simulink model "Vector_control_10Hp_with_20usec"  (R2014a)
settings: Solver=ode5  StartTime=0.0  StopTime=10  FixedStep=20e-6  RelTol=1e-3
InitFcn:
  | Lr=0.1241+0.003045;
  | Lm=0.1241;
  | Ls=0.1241+0.003045;
undefined symbols (not defined in the file): DiscIntNeverNeededParam, driveGuiManager, gcbh, sps_rtmsupport, Ts
libraries: powerlib x10, powerlib_meascontrol x5, simulink_extras x4, AC3DriveInternalModels x2, DriveInternalModels x1, simulink x1
settings Model: Creator=Bharat  LastModifiedBy=apple
settings DebuggingCC: UnderspecifiedInitializationDetection=Classic  StateNameClashWarn=warning

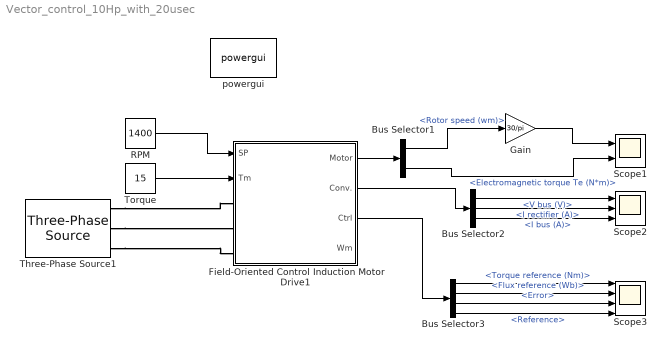
== system Vector_control_10Hp_with_20usec ==
  Bus Selector1 : BusSelector  OutputSignals=Mechanical.Rotor speed (wm),Mechanical.Electromagnetic torque Te (N*m)
  Bus Selector2 : BusSelector  OutputSignals=V bus (V),I rectifier (A),I bus (A)
  Bus Selector3 : BusSelector  OutputSignals=Torque reference (Nm),Flux reference (Wb),Error,Reference
  Field-Oriented Control Induction Motor Drive1 : Subsystem  LoadFcn=sps_rtmsupport('LoadFcn',gcbh); driveGuiManager('Load',get_param(gcb,'driveType'), gcbh);  StartFcn=sps_rtmsupport('StartFcn',gcbh);  StopFcn=|  mask(Field-Oriented Control Induction Motor Drive){showMaskWarnings=on, AverageValue=off, MechanicalLoad=Torque Tm, driveType=AC3, outputBusMode=Multiple output buses}
      | sps_rtmsupport('StopFcn',gcbh);                                   
      | %driveGuiManager('ReactivateGui',get_param(gcb,'driveType'),gcbh);
      mask prompts: showMaskWarnings "Show mask synchronization warnings"; AverageValue "Average value model"; MechanicalLoad "Mechanical input:"; driveType "Drive type"; outputBusMode "Output bus mode:"
      mask init:
      | block=gcb;
      | [X1,X1m,X2,X2m,X3,X4,Y1,Y1m,Y2,Y2m,Y3,Y4,color1,color2,INp,OUTp,Ts,machineType] = spsDrivesMaskInit(block,driveType,AverageValue);
      | %spsDrivesOutputSelectorCbak(block);
      settings: CopyFcn=sps_rtmsupport('CopyFcn',gcbh);  DeleteFcn="sps_rtmsupport('DeleteFcn',gcbh); driveGuiManager('Delete',get_param(gcb,'driveType')  ,gcbh)"  UndoDeleteFcn=sps_rtmsupport('UndoDeleteFcn',gcbh);  ModelCloseFcn=sps_rtmsupport('ModelCloseFcn',gcbh);  PreSaveFcn=sps_rtmsupport('PreSaveFcn',gcbh);  PostSaveFcn=sps_rtmsupport('PostSaveFcn',gcbh);  NameChangeFcn=sps_rtmsupport('NameChangeFcn',gcbh);  PreCopyFcn=sps_rtmsupport('PreCopyFcn',gcbh);  CloseFcn="sps_rtmsupport('CloseFcn',gcbh); %driveGuiManager('Delete',get_param(gcb,'driveType')  ,gcbh)"  PreDeleteFcn=sps_rtmsupport('PreDeleteFcn',gcbh);  ParentCloseFcn="driveGuiManager('Hide',get_param(gcb,'driveType')  ,gcbh)"
      settings: OpenFcn=|
      | sps_rtmsupport('parametereditingmodes',gcbh, [1 2 3 4 5]); if (power_openblockproxy ('secondary'))
      | driveGuiManager('Create',get_param(gcb,'driveType')  ,gcbh)
      | end;
      mask Help: helpview(psbhelp)
      mask TypeOptions MechanicalLoad: Torque Tm | Speed w | Mechanical rotational port
      mask TypeOptions driveType: AC3
      mask TypeOptions outputBusMode: Multiple output buses | Single output bus
      mask Display:
      | patch([X1 X1m],[Y1 Y1m],color1);
      | patch(X3,Y3,color2);
      | plot([X1 X1m X2 X2m X3 X4],[Y1 Y1m Y2 Y2m Y3 Y4]);
      | text(0.5,0.3,'AC3','HorizontalAlignment','center')
      | HaveSPSMec = (strcmp(MechanicalLoad,'Torque Tm') || strcmp(MechanicalLoad,'Speed w'));
      | if (HaveSPSMec==1 && strcmp(outputBusMode,'Multiple output buses'))
      |     port_label('input',2,INp)
      |     port_label('output',4,OUTp)
      | end
      | if (HaveSPSMec==1 && strcmp(outputBusMode,'Single output bus'))
      |     port_label('input',2,INp)
      |     port_label('output',2,OUTp)
      | end
  Gain : Gain  Gain=30/pi
  RPM : Constant  Value=1400
  Scope1 : Scope  NumInputPorts=2
      settings: YMin=1399.8~5  YMax=1402~20
  Scope2 : Scope  NumInputPorts=3
      settings: YMin=215~3.5~-22.5  YMax=262.5~12.5~22.5
  Scope3 : Scope  NumInputPorts=4
      settings: YMin=104.765~5.75~-5~-5  YMax=104.83~10.75~5~5  SaveName=ScopeData2
  Three-Phase Source1 : powerlib/Electrical Sources/Three-Phase Source  Voltage=400  PhaseAngle=0  Frequency=50  InternalConnection=Yg  SpecifyImpedance=on  Resistance=0.8929  Inductance=16.58e-3  ShortCircuitLevel=100e6  BaseVoltage=25e3  XRratio=7  BusType=swing  Pref=0  Qref=0  Qmin=-inf  Qmax=inf
  Torque : Constant  Value=15
  powergui : powerlib/powergui  Priority=1  SimulationMode=Discrete  SolverType=Backward Euler  SampleTime=20e-6  frequency=60  SPID=off  DisableSnubberDevices=off  DisableRonSwitches=off  DisableVfSwitches=off  SwTol=0  Interpol=off  DisplayEquations=off  Ts=0  methode=off  frequencyindice=50  Pbase=100e6  ErrMax=1e-4  Iterations=50  UnitsV=kV  UnitsW=MW  FunctionMessages=off  echomessages=off  HookPort=off  EnableUseOfTLC=off  x0status=blocks  RestoreLinks=warning  ResistiveCurrentMeasurement=off  Frange=[0:2:500]  Ylog=off  Xlog=on  ShowGrid=off  save=off  variable=ZData  structure=0  ZoomFFT=off  StartTime=0.0  cycles=1  DisplayStyle=1  fundamental=60  FreqAxis=off  MaxFrequency=1000  frequencyindicesteady=1  RmsSteady=1  display=off
  wires:
  RPM/1 -> Field-Oriented Control Induction Motor Drive1/1(SP)
  Torque/1 -> Field-Oriented Control Induction Motor Drive1/2(Tm)
  Field-Oriented Control Induction Motor Drive1/1(Motor) -> Bus Selector1/1
  Bus Selector1/1 -> Gain/1  "<Rotor speed (wm)>"
  Bus Selector1/2 -> Scope1/2  "<Electromagnetic torque Te (N*m)>"
  Field-Oriented Control Induction Motor Drive1/2(Conv.) -> Bus Selector2/1
  Bus Selector2/1 -> Scope2/1  "<V bus (V)>"
  Bus Selector2/2 -> Scope2/2  "<I rectifier (A)>"
  Field-Oriented Control Induction Motor Drive1/3(Ctrl) -> Bus Selector3/1
  Bus Selector3/1 -> Scope3/1  "<Torque reference (Nm)>"
  Bus Selector3/2 -> Scope3/2  "<Flux reference (Wb)>"
  Bus Selector2/3 -> Scope2/3  "<I bus (A)>"
  Bus Selector3/3 -> Scope3/3  "<Error>"
  Bus Selector3/4 -> Scope3/4  "<Reference>"
  Gain/1 -> Scope1/1
  connections:
  Three-Phase Source1/RConn2 -- Field-Oriented Control Induction Motor Drive1/LConn2
  Three-Phase Source1/RConn3 -- Field-Oriented Control Induction Motor Drive1/LConn3
  Three-Phase Source1/RConn1 -- Field-Oriented Control Induction Motor Drive1/LConn1

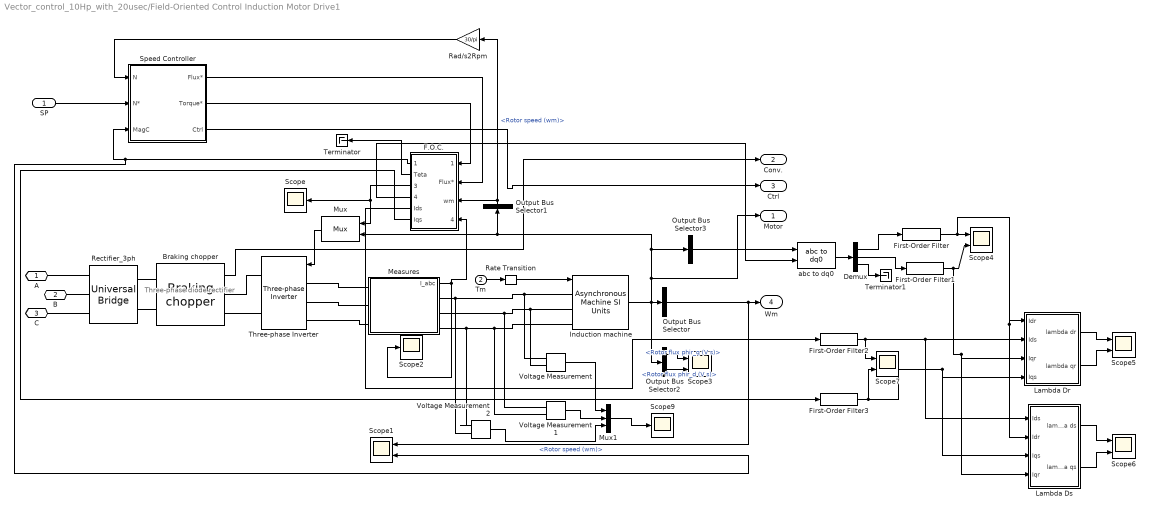
== system Vector_control_10Hp_with_20usec/Field-Oriented Control Induction Motor Drive1 ==
  note: Three-phase
      | diode rectifier
  SP : Inport
  Tm : Inport  Port=2
  Braking chopper : DriveInternalModels/AC drives/Braking chopper  chopa=500  chopd=490  freq_chop=4000  cap_bus=2000e-6  br=8
  Demux : Demux  Outputs=3
  F.O.C. : Subsystem  mask(FOC){freq_max=20000, in_flux=0.45, Lm=0.1722, Rr=1.395, Llr=0.005839, p=2, h=0.1, kp=40, ki=50, fc=16, csat=[-2,2], Tvect=20e-6}
      mask prompts: freq_max "Maximum inverter frequency (Hz)"; in_flux "Initial machine flux (Wb)"; Lm "Motor mutual inductance (H)"; Rr "Motor rotor resistance (ohms)"; Llr "Motor rotor leakage inductance (H)"; p "Motor pairs of poles"; h "Current regulator - current hysteresis bandwidth (A)"; kp "Flux controller - proportional gain"; ki "Flux controller - integral gain"; fc "Flux controller - flux estimation low-pass filter cutoff frequency (Hz)"; csat "Flux controller - controller output flux saturation (Wb) [negative,positive]"; Tvect "Vector control sampling time (s)"
      mask help: This block implements a field oriented controller.
      mask init:
      | Lr=Lm+Llr;
      | [X1,X1m,X2,X2m,X3,X4,Y1,Y1m,Y2,Y2m,Y3,Y4,color1,color2]=spsdrivelogo;
      mask Display:
      | patch([X1 X1m],[Y1 Y1m],color1);
      | patch(X3,Y3,color2);
      | plot([X1 X1m X2 X2m X3 X4],[Y1 Y1m Y2 Y2m Y3 Y4]);
  First-Order Filter : powerlib_meascontrol/Filters/First-Order Filter  FilterType=Lowpass  Tc=1/100  Ts=0  Initialize=on  Vac_Init=[0, 0, 60]  Vdc_Init=0  PlotResponse=off  FreqRange="[0,  200,  1]"
  First-Order Filter1 : powerlib_meascontrol/Filters/First-Order Filter  FilterType=Lowpass  Tc=1/100  Ts=0  Initialize=on  Vac_Init=[0, 0, 60]  Vdc_Init=0  PlotResponse=off  FreqRange="[0,  200,  1]"
  First-Order Filter2 : powerlib_meascontrol/Filters/First-Order Filter  FilterType=Lowpass  Tc=1/200  Ts=0  Initialize=on  Vac_Init=[0, 0, 60]  Vdc_Init=0  PlotResponse=off  FreqRange="[0,  200,  1]"
  First-Order Filter3 : powerlib_meascontrol/Filters/First-Order Filter  FilterType=Lowpass  Tc=1/200  Ts=0  Initialize=on  Vac_Init=[0, 0, 60]  Vdc_Init=0  PlotResponse=off  FreqRange="[0,  200,  1]"
  Induction machine : powerlib/Machines/Asynchronous Machine SI Units  PresetModel="16:  10 HP (7.5KW)  400 V 50Hz 1440 RPM"  MechanicalLoad=Torque Tm  ShowDetailedParameters=on  RotorType=Squirrel-cage  ReferenceFrame=Rotor  Units=SI  MeasurementBus=off  NominalParameters=[7500 400 50]  Stator=[0.7384 0.003045]  Rotor=[0.7402 0.003045]  Cage1=[ 0.022 0.226/377]  Cage2=[ 0.022 0.226/377]  Lm=0.1241  Mechanical=[0.0343 0.000503 2]  PolePairs=2  InitialConditions=[1,0,0,0,0,0,0,0]  SimulateSaturation=off  Saturation=[0 0;0 0]  LoadFlowParameters=0  TsPowergui=0  TsBlock=-1  IterativeModel=Forward Euler  Pmec=0
  Lambda Dr : Subsystem
  Lambda Ds : Subsystem
  Measures : Subsystem
  Mux : AC3DriveInternalModels/Mux
  Mux1 : Mux  Inputs=3
  Output Bus Selector : BusSelector  OutputSignals=Mechanical.Rotor speed (wm)
  Output Bus Selector1 : BusSelector  OutputSignals=Mechanical.Rotor speed (wm)
  Output Bus Selector2 : BusSelector  OutputSignals=Rotor measurements.Rotor flux phir_q (V s),Rotor measurements.Rotor flux phir_d (V s)
  Output Bus Selector3 : BusSelector  OutputSignals=Rotor measurements.Rotor current ir_a (A),Rotor measurements.Rotor current ir_b (A),Rotor measurements.Rotor current ir_c (A)  OutputAsBus=on
  Rad/s2Rpm : Gain  Gain=30/pi  SaturateOnIntegerOverflow=on  OutDataTypeStr=Inherit: Same as input  ParamDataTypeStr=Inherit: Same as input
  Rate Transition : RateTransition  OutPortSampleTime=Ts
  Rectifier_3ph : powerlib/Power Electronics/Universal Bridge  Arms=3  SnubberResistance=10e3  SnubberCapacitance=20e-9  Device=Diodes  Ron=1e-3  Lon=0  ForwardVoltages="[  0,  0  ]"  ForwardVoltage=1.3  GTOparameters=[ 10e-6, 20e-6 ]  IGBTparameters=[ 1e-6 , 2e-6 ]  Measurements=All voltages and currents  Measurements_2=None  converterType=Rectifier
  Scope : Scope
      settings: SaveName=ScopeData4
  Scope{1,3..7} (6 alike) : Scope  NumInputPorts=2
      Scope1 settings: YMin=32~0.95  YMax=53~1.05  SaveName=ScopeData5
      Scope3 settings: YMin=-5~-5  YMax=5~5  SaveName=ScopeData10
      Scope4 settings: YMin=0.04~-18.025  YMax=0.19~-17.825  SaveName=ScopeData11
      Scope5 settings: YMin=-2.5~-10  YMax=5~12  SaveName=ScopeData13
      Scope6 settings: YMin=-2.5~-10  YMax=5~12  SaveName=ScopeData14
      Scope7 settings: YMin=0.04~-18.025  YMax=0.19~-17.825  SaveName=ScopeData15
  Scope2 : Scope
      settings: SaveName=ScopeData8
  Scope9 : Scope
      settings: SaveName=ScopeData21
  Speed Controller : Subsystem  mask(Speed controller){SwK=Speed regulation, fn=50, ramp=[-1500,1500], kp=0.9, ki=6.4, fc=100, ctrl_sat=[-28,28], p=2, nf=0.45, Tsc=100e-6}
      mask prompts: SwK "Regulation type"; fn "Machine nominal frequency (Hz)"; ramp "Speed reference ramp  (rpm/s) [deceleration,acceleration]"; kp "Proportional gain"; ki "Integral gain"; fc "Speed measurement - low-pass filter cutoff frequency (Hz)"; ctrl_sat "Controller output torque saturation (N.m) [negative,positive]"; p "Motor pairs of poles"; nf "Machine nominal flux (Wb)"; Tsc "Controller sampling time (s)"
      mask help: This block implements a PI speed regulator.
      mask init:
      | bs=2*30*fn/p;
      | [X1,X1m,X2,X2m,X3,X4,Y1,Y1m,Y2,Y2m,Y3,Y4,color1,color2]=spsdrivelogo;
      | if SwK == 1
      |     set_param(gcb,'MaskVisibilities',{'on','on','on','on','on','on','on','on','on','on'})
      | else
      |     set_param(gcb,'MaskVisibilities',{'on','on','off','off','off','off','on','on','on','on'})
      | end
      mask TypeOptions SwK: Speed regulation | Torque regulation
      mask Display:
      | patch([X1 X1m],[Y1 Y1m],color1);
      | patch(X3,Y3,color2);
      | plot([X1 X1m X2 X2m X3 X4],[Y1 Y1m Y2 Y2m Y3 Y4]);
  Terminator : Terminator
  Terminator1 : Terminator
  Three-phase Inverter : AC3DriveInternalModels/Three-phase Inverter  Arms=3  SnubberResistance=5e3  SnubberCapacitance=inf  Device=IGBT / Diodes  Ron=1e-3  Lon=0  ForwardVoltages=[0.8,0.8]  ForwardVoltage=0  GTOparameters=[10e-6,20e-6]  IGBTParameters=[1e-6,2e-6]  Measurements=All voltages and currents  converterType=Inverter  SourceFrequency=60  Stator=[1.405,0.005839]  Rotor=[1.395,0.005839]  Lm=0.1722  p=2  ReferenceFrame=Rotor
  Voltage Measurement : powerlib/Measurements/Voltage Measurement  PhasorSimulation=off  OutputType=Complex  PSBequivalent=0
  Voltage Measurement1 : powerlib/Measurements/Voltage Measurement  PhasorSimulation=off  OutputType=Complex  PSBequivalent=0
  Voltage Measurement2 : powerlib/Measurements/Voltage Measurement  PhasorSimulation=off  OutputType=Complex  PSBequivalent=0
  abc to dq0 : powerlib_meascontrol/Transformations/abc to dq0  Alignment=Aligned with phase A axis
  A : PMIOPort  Port=1  Side=Left
  B : PMIOPort  Port=2  Side=Left
  C : PMIOPort  Port=3  Side=Left
  Motor : Outport
  Conv. : Outport  Port=2
  Ctrl : Outport  Port=3
  Wm : Outport  Port=4
  wires:
  Induction machine/1 -> Motor/1, Output Bus Selector3/1, Mux/2, Output Bus Selector1/1, Output Bus Selector2/1, Output Bus Selector/1
  Measures/1(I_abc) -> F.O.C./4(I_ABC), Scope2/1
  F.O.C./2(Teta) -> Terminator/1
  Speed Controller/3(Ctrl) -> Ctrl/1
  Speed Controller/1(Flux*) -> F.O.C./2(Flux*)
  Speed Controller/2(Torque*) -> F.O.C./1(Torque*)
  Rad/s2Rpm/1 -> Speed Controller/1(N)
  Braking chopper/1 -> Conv./1
  F.O.C./3(Gates) -> Mux/1, Scope/1
  Mux/1 -> Three-phase Inverter/1
  Output Bus Selector/1 -> Scope1/1, Wm/1  "<Rotor speed (wm)>"
  Tm/1 -> Rate Transition/1
  Rate Transition/1 -> Induction machine/1
  F.O.C./1(MagC) -> Scope1/2, Speed Controller/3(MagC)
  Output Bus Selector2/1 -> Scope3/1  "<Rotor flux phir_q (V s)>"
  Output Bus Selector2/2 -> Scope3/2  "<Rotor flux phir_d (V s)>"
  Output Bus Selector3/1 -> abc to dq0/1
  F.O.C./4(Teta1) -> abc to dq0/2
  abc to dq0/1 -> Demux/1
  Demux/1 -> First-Order Filter/1
  Demux/2 -> First-Order Filter1/1
  Demux/3 -> Terminator1/1
  First-Order Filter/1 -> Lambda Ds/2(Idr), Lambda Dr/1(Idr), Scope4/1
  First-Order Filter1/1 -> Lambda Ds/4(Iqr), Lambda Dr/3(Iqr), Scope4/2
  Lambda Dr/1(lambda dr) -> Scope5/1
  Lambda Dr/2(lambda qr) -> Scope5/2
  Lambda Ds/1(lambda ds) -> Scope6/1
  Lambda Ds/2(lambda qs) -> Scope6/2
  F.O.C./5(Ids) -> First-Order Filter2/1
  F.O.C./6(Iqs) -> First-Order Filter3/1
  First-Order Filter3/1 -> Scope7/2, Lambda Ds/3(Iqs), Lambda Dr/4(Iqs)
  First-Order Filter2/1 -> Scope7/1, Lambda Ds/1(Ids), Lambda Dr/2(Ids)
  SP/1 -> Speed Controller/2(N*)
  Voltage Measurement/1 -> Mux1/1
  Voltage Measurement1/1 -> Mux1/2
  Voltage Measurement2/1 -> Mux1/3
  Mux1/1 -> Scope9/1
  Output Bus Selector1/1 -> Rad/s2Rpm/1, F.O.C./3(wm)  "<Rotor speed (wm)>"
  connections:
  Measures/RConn1 -- Voltage Measurement2/LConn2 -- Voltage Measurement/LConn1 -- Induction machine/LConn1
  Measures/RConn2 -- Voltage Measurement1/LConn1 -- Voltage Measurement/LConn2 -- Induction machine/LConn2
  Measures/RConn3 -- Voltage Measurement2/LConn1 -- Voltage Measurement1/LConn2 -- Induction machine/LConn3
  Three-phase Inverter/LConn1 -- Measures/LConn1
  Three-phase Inverter/LConn2 -- Measures/LConn2
  Three-phase Inverter/LConn3 -- Measures/LConn3
  Braking chopper/RConn1 -- Three-phase Inverter/RConn1
  Braking chopper/RConn2 -- Three-phase Inverter/RConn2
  Braking chopper/LConn1 -- Rectifier_3ph/RConn1
  Braking chopper/LConn2 -- Rectifier_3ph/RConn2
  A/RConn1 -- Rectifier_3ph/LConn1
  B/RConn1 -- Rectifier_3ph/LConn2
  C/RConn1 -- Rectifier_3ph/LConn3

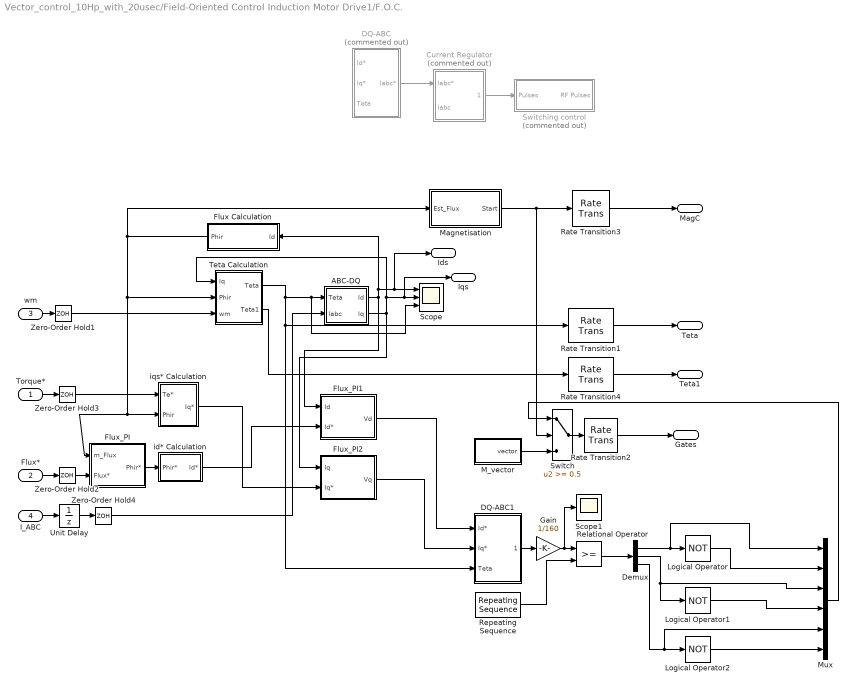
== system Vector_control_10Hp_with_20usec/Field-Oriented Control Induction Motor Drive1/F.O.C. ==
  Torque* : Inport
  Flux* : Inport  Port=2
  wm : Inport  Port=3
  I_ABC : Inport  Port=4
  ABC-DQ : Subsystem
  Current Regulator : Subsystem  Commented=on
  DQ-ABC : Subsystem  Commented=on
  DQ-ABC1 : Subsystem
  Demux : Demux  Outputs=3
  Flux Calculation : Subsystem  mask(Flux Calcultation){}
      mask init:
      | NF=0.44572610323020e-6;
      | DF=[1 -0.99998715486734];
  Flux_PI : Subsystem
  Flux_PI1 : Subsystem
  Flux_PI2 : Subsystem
  Gain : Gain  Gain=1/160
  Logical Operator : Logic  Operator=NOT  AllPortsSameDT=off  OutDataTypeStr=boolean
  Logical Operator1 : Logic  Operator=NOT  AllPortsSameDT=off  OutDataTypeStr=boolean
  Logical Operator2 : Logic  Operator=NOT  AllPortsSameDT=off  OutDataTypeStr=boolean
  M_vector : Subsystem
  Magnetisation : Subsystem
  Mux : Mux  Inputs=6
  Rate Transition1 : RateTransition  OutPortSampleTime=Ts
  Rate Transition2 : RateTransition
  Rate Transition3 : RateTransition
  Rate Transition4 : RateTransition  OutPortSampleTime=Ts
  Relational Operator : RelationalOperator  OutDataTypeStr=boolean
  Repeating Sequence : simulink/Sources/Repeating Sequence  rep_seq_t=[0 1/8000 1/4000 3/8000 1/2000]  rep_seq_y=[0 1 0 -1 0]
  Scope : Scope  NumInputPorts=3
      settings: YMin=1.5~17.5~2.5  YMax=7~22.25~35  SaveName=ScopeData3
  Scope1 : Scope
      settings: YMin=-3  YMax=3  SaveName=ScopeData12
  Switch : Switch  Threshold=0.5  SaturateOnIntegerOverflow=on
  Switching control : Subsystem  Commented=on
  Teta Calculation : Subsystem
  Unit Delay : UnitDelay  SampleTime=-1
  Zero-Order Hold{1..4} (4 alike) : ZeroOrderHold  SampleTime=Tvect
  id* Calculation : Subsystem
  iqs* Calculation : Subsystem
  MagC : Outport
  Teta : Outport  Port=2
  Gates : Outport  Port=3
  Teta1 : Outport  Port=4
  Ids : Outport  Port=5
  Iqs : Outport  Port=6
  wires:
  Zero-Order Hold2/1 -> Flux_PI/2(Flux*)
  ABC-DQ/1(Id) -> Ids/1, Scope/1, Flux Calculation/1(Id), Flux_PI1/1(Id)
  ABC-DQ/2(Iq) -> Flux_PI2/1(Iq), Teta Calculation/1(Iq), Iqs/1, Scope/2
  Flux Calculation/1(Phir) -> Magnetisation/1(Est_Flux), Teta Calculation/2(Phir), Flux_PI/1(m_Flux), iqs* Calculation/2(Phir)
  iqs* Calculation/1(Iq*) -> Flux_PI2/2(Iq*)
  id* Calculation/1(Id*) -> Flux_PI1/2(Id*)
  I_ABC/1 -> Unit Delay/1
  wm/1 -> Zero-Order Hold1/1
  Current Regulator/1(Pulses) -> Switching control/1(Pulses)
  Torque*/1 -> Zero-Order Hold3/1
  Flux*/1 -> Zero-Order Hold2/1
  DQ-ABC/1(Iabc*) -> Current Regulator/1(Iabc*)
  Switch/1 -> Rate Transition2/1
  Magnetisation/1(Start) -> Switch/2, Rate Transition3/1
  M_vector/1(vector) -> Switch/3
  Rate Transition2/1 -> Gates/1
  Rate Transition3/1 -> MagC/1
  Rate Transition1/1 -> Teta/1
  Zero-Order Hold3/1 -> iqs* Calculation/1(Te*)
  Zero-Order Hold4/1 -> ABC-DQ/2(Iabc)
  Zero-Order Hold1/1 -> Teta Calculation/3(wm)
  Flux_PI/1(Phir*) -> id* Calculation/1(Phir*)
  Unit Delay/1 -> Zero-Order Hold4/1
  Teta Calculation/2(Teta1) -> Rate Transition4/1
  Rate Transition4/1 -> Teta1/1
  Teta Calculation/1(Teta) -> Scope/3, ABC-DQ/1(Teta), DQ-ABC1/3(Teta), Rate Transition1/1
  Flux_PI2/1(Vq) -> DQ-ABC1/2(Iq*)
  Flux_PI1/1(Vd) -> DQ-ABC1/1(Id*)
  DQ-ABC1/1(Vabc*) -> Gain/1
  Repeating Sequence/1 -> Relational Operator/2
  Relational Operator/1 -> Demux/1
  Demux/1 -> Mux/1, Logical Operator/1
  Demux/3 -> Mux/5, Logical Operator2/1
  Logical Operator/1 -> Mux/2
  Demux/2 -> Logical Operator1/1, Mux/3
  Logical Operator1/1 -> Mux/4
  Logical Operator2/1 -> Mux/6
  Mux/1 -> Switch/1
  Gain/1 -> Scope1/1, Relational Operator/1

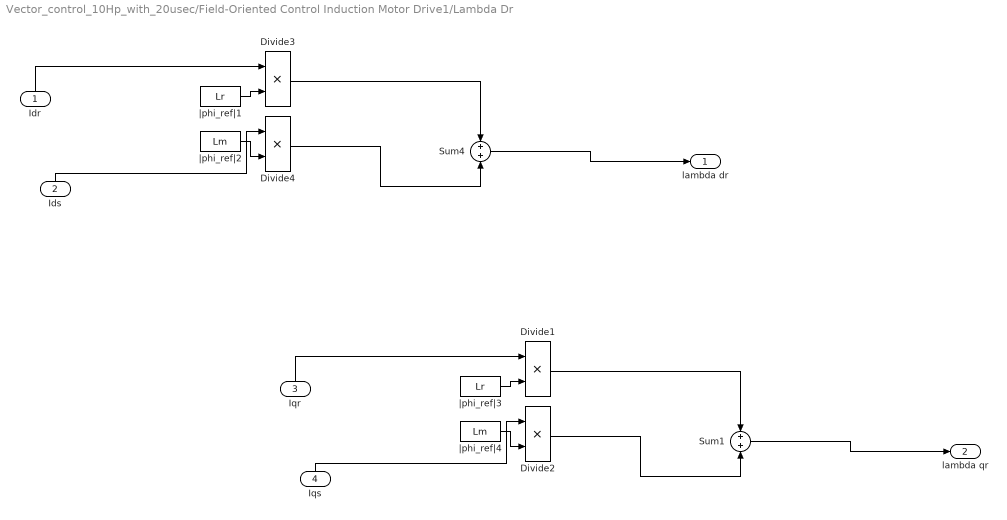
== system Vector_control_10Hp_with_20usec/Field-Oriented Control Induction Motor Drive1/Lambda Dr ==
  Idr : Inport
  Ids : Inport  Port=2
  Iqr : Inport  Port=3
  Iqs : Inport  Port=4
  Divide{1..4} (4 alike) : Product
  Sum1 : Sum
  Sum4 : Sum
  |phi_ref|1 : Constant  Value=Lr
  |phi_ref|2 : Constant  Value=Lm
  |phi_ref|3 : Constant  Value=Lr
  |phi_ref|4 : Constant  Value=Lm
  lambda dr : Outport
  lambda qr : Outport  Port=2
  wires:
  Ids/1 -> Divide4/1
  Idr/1 -> Divide3/1
  |phi_ref|1/1 -> Divide3/2
  |phi_ref|2/1 -> Divide4/2
  Divide3/1 -> Sum4/1
  Divide4/1 -> Sum4/2
  Sum4/1 -> lambda dr/1
  Iqs/1 -> Divide2/1
  Iqr/1 -> Divide1/1
  |phi_ref|3/1 -> Divide1/2
  |phi_ref|4/1 -> Divide2/2
  Divide1/1 -> Sum1/1
  Divide2/1 -> Sum1/2
  Sum1/1 -> lambda qr/1

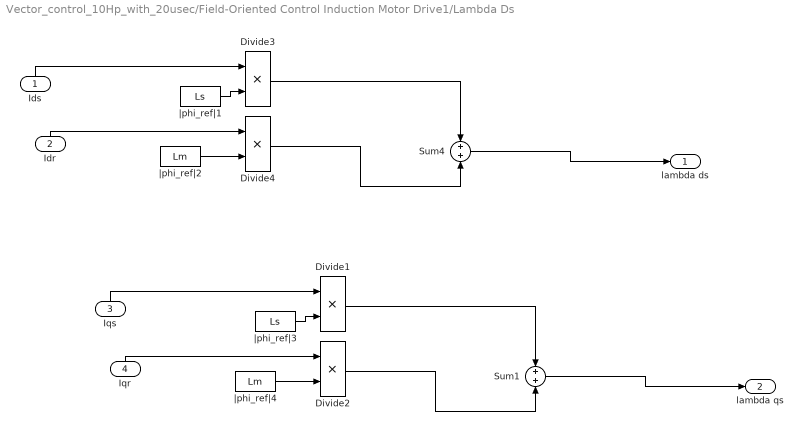
== system Vector_control_10Hp_with_20usec/Field-Oriented Control Induction Motor Drive1/Lambda Ds ==
  Ids : Inport
  Idr : Inport  Port=2
  Iqs : Inport  Port=3
  Iqr : Inport  Port=4
  Divide{1..4} (4 alike) : Product
  Sum1 : Sum
  Sum4 : Sum
  |phi_ref|1 : Constant  Value=Ls
  |phi_ref|2 : Constant  Value=Lm
  |phi_ref|3 : Constant  Value=Ls
  |phi_ref|4 : Constant  Value=Lm
  lambda ds : Outport
  lambda qs : Outport  Port=2
  wires:
  Sum4/1 -> lambda ds/1
  Divide4/1 -> Sum4/2
  Divide3/1 -> Sum4/1
  |phi_ref|2/1 -> Divide4/2
  |phi_ref|1/1 -> Divide3/2
  Ids/1 -> Divide3/1
  Idr/1 -> Divide4/1
  Sum1/1 -> lambda qs/1
  Divide2/1 -> Sum1/2
  Divide1/1 -> Sum1/1
  |phi_ref|4/1 -> Divide2/2
  |phi_ref|3/1 -> Divide1/2
  Iqs/1 -> Divide1/1
  Iqr/1 -> Divide2/1

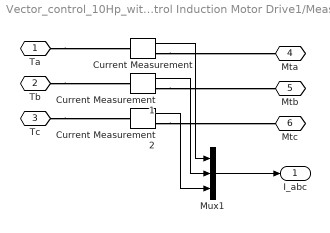
== system Vector_control_10Hp_with_20usec/Field-Oriented Control Induction Motor Drive1/Measures ==
  Current Measurement : powerlib/Measurements/Current Measurement  Tag=PoWeRsYsTeMmEaSuReMeNt  PhasorSimulation=off  OutputType=Complex  PSBequivalent=0
  Current Measurement1 : powerlib/Measurements/Current Measurement  Tag=PoWeRsYsTeMmEaSuReMeNt  PhasorSimulation=off  OutputType=Complex  PSBequivalent=0
  Current Measurement2 : powerlib/Measurements/Current Measurement  Tag=PoWeRsYsTeMmEaSuReMeNt  PhasorSimulation=off  OutputType=Complex  PSBequivalent=0
  Mux1 : Mux  Inputs=3
  Ta : PMIOPort  Port=1  Side=Left
  Tb : PMIOPort  Port=2  Side=Left
  Tc : PMIOPort  Port=3  Side=Left
  Mta : PMIOPort  Port=4  Side=Right
  Mtb : PMIOPort  Port=5  Side=Right
  Mtc : PMIOPort  Port=6  Side=Right
  I_abc : Outport
  wires:
  Mux1/1 -> I_abc/1
  Current Measurement1/1 -> Mux1/2
  Current Measurement/1 -> Mux1/1
  Current Measurement2/1 -> Mux1/3
  connections:
  Current Measurement1/RConn1 -- Mtb/RConn1
  Tb/RConn1 -- Current Measurement1/LConn1
  Current Measurement/RConn1 -- Mta/RConn1
  Ta/RConn1 -- Current Measurement/LConn1
  Tc/RConn1 -- Current Measurement2/LConn1
  Current Measurement2/RConn1 -- Mtc/RConn1

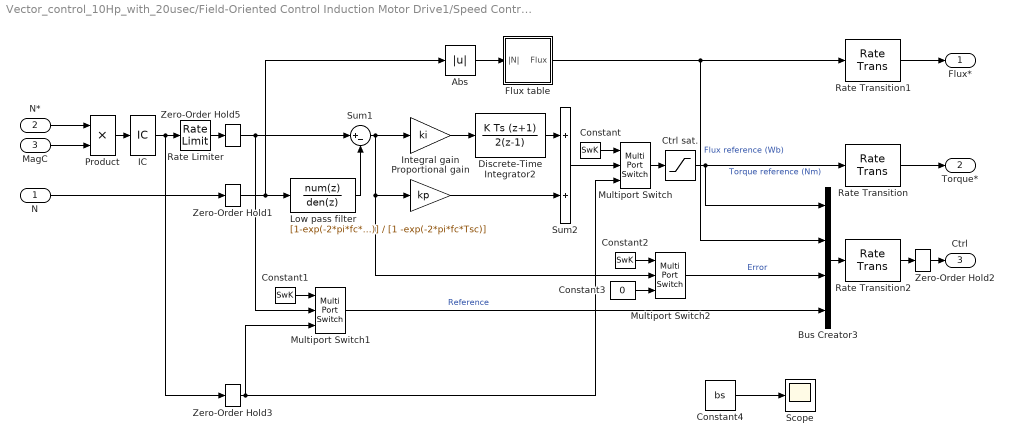
== system Vector_control_10Hp_with_20usec/Field-Oriented Control Induction Motor Drive1/Speed Controller ==
  N : Inport
  N* : Inport  Port=2
  MagC : Inport  Port=3
  Abs : Abs  SaturateOnIntegerOverflow=on
  Bus Creator3 : BusCreator
  Constant : Constant  Value=SwK
  Constant1 : Constant  Value=SwK
  Constant2 : Constant  Value=SwK
  Constant3 : Constant  Value=0
  Constant4 : Constant  Value=bs
  Ctrl sat. : Saturate  UpperLimit=ctrl_sat(2)  LowerLimit=ctrl_sat(1)
  Discrete-Time Integrator2 : DiscreteIntegrator  IntegratorMethod=Integration: Trapezoidal  SampleTime=Tsc  LimitOutput=on  UpperSaturationLimit=ctrl_sat(2)  LowerSaturationLimit=ctrl_sat(1)  ICPrevOutput=DiscIntNeverNeededParam  ICPrevScaledInput=DiscIntNeverNeededParam
  Flux table : Subsystem
      mask Display: plot([0;1800;2000;2500;3000;3500], [1;1;0.90*1;0.72*1;0.6*1;0.51*1])
  IC : InitialCondition  Value=0
  Integral gain : Gain  Gain=ki  SaturateOnIntegerOverflow=on  OutDataTypeStr=Inherit: Same as input  ParamDataTypeStr=Inherit: Same as input
  Low pass filter : DiscreteTransferFcn  Numerator=[1-exp(-2*pi*fc*Tsc)]  Denominator=[1 -exp(-2*pi*fc*Tsc)]  SampleTime=Tsc
  Multiport Switch : MultiPortSwitch  Inputs=2  SaturateOnIntegerOverflow=on
  Multiport Switch1 : MultiPortSwitch  Inputs=2  SaturateOnIntegerOverflow=on
  Multiport Switch2 : MultiPortSwitch  Inputs=2  SaturateOnIntegerOverflow=on
  Product : Product  SaturateOnIntegerOverflow=on  OutDataTypeStr=Inherit: Same as first input
  Proportional gain : Gain  Gain=kp  SaturateOnIntegerOverflow=on  OutDataTypeStr=Inherit: Same as input  ParamDataTypeStr=Inherit: Same as input
  Rate Limiter : RateLimiter  RisingSlewLimit=ramp(2)  FallingSlewLimit=ramp(1)  LinearizeAsGain=off
  Rate Transition : RateTransition
  Rate Transition1 : RateTransition
  Rate Transition2 : RateTransition
  Scope : Scope
      settings: YMin=1800  YMax=1800  SaveName=ScopeData9
  Sum1 : Sum  Inputs=|+-  SaturateOnIntegerOverflow=on  InputSameDT=on  OutDataTypeStr=Inherit: Same as first input
  Sum2 : Sum  SaturateOnIntegerOverflow=on  InputSameDT=on  OutDataTypeStr=Inherit: Same as first input
  Zero-Order Hold1 : ZeroOrderHold  SampleTime=Tsc
  Zero-Order Hold2 : ZeroOrderHold  SampleTime=Ts
  Zero-Order Hold3 : ZeroOrderHold  SampleTime=Tsc
  Zero-Order Hold5 : ZeroOrderHold  SampleTime=Tsc
  Flux* : Outport
  Torque* : Outport  Port=2
  Ctrl : Outport  Port=3
  wires:
  Constant3/1 -> Multiport Switch2/3
  Constant2/1 -> Multiport Switch2/1
  Multiport Switch2/1 -> Bus Creator3/3  "Error"
  Multiport Switch1/1 -> Bus Creator3/4  "Reference"
  Zero-Order Hold3/1 -> Multiport Switch1/3, Multiport Switch/3
  Constant1/1 -> Multiport Switch1/1
  Sum2/1 -> Multiport Switch/2
  Constant/1 -> Multiport Switch/1
  Multiport Switch/1 -> Ctrl sat./1
  Zero-Order Hold5/1 -> Multiport Switch1/2, Sum1/1
  Rate Limiter/1 -> Zero-Order Hold5/1
  MagC/1 -> Product/2
  Product/1 -> IC/1
  N*/1 -> Product/1
  Low pass filter/1 -> Sum1/2
  Zero-Order Hold2/1 -> Ctrl/1
  Bus Creator3/1 -> Rate Transition2/1
  Rate Transition2/1 -> Zero-Order Hold2/1
  Zero-Order Hold1/1 -> Low pass filter/1, Abs/1
  IC/1 -> Zero-Order Hold3/1, Rate Limiter/1
  Rate Transition1/1 -> Flux*/1
  Rate Transition/1 -> Torque*/1
  Flux table/1(Flux) -> Bus Creator3/2, Rate Transition1/1  "Flux reference (Wb)"
  Abs/1 -> Flux table/1(|N|)
  Proportional gain/1 -> Sum2/2
  Discrete-Time Integrator2/1 -> Sum2/1
  N/1 -> Zero-Order Hold1/1
  Sum1/1 -> Multiport Switch2/2, Proportional gain/1, Integral gain/1
  Integral gain/1 -> Discrete-Time Integrator2/1
  Ctrl sat./1 -> Bus Creator3/1, Rate Transition/1  "Torque reference (Nm)"
  Constant4/1 -> Scope/1

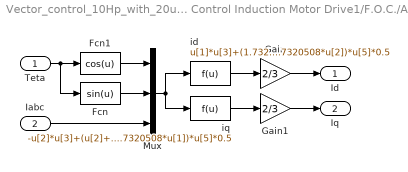
== system Vector_control_10Hp_with_20usec/Field-Oriented Control Induction Motor Drive1/F.O.C./ABC-DQ ==
  Teta : Inport
  Iabc : Inport  Port=2
  Fcn : Fcn  Expr=sin(u)
  Fcn1 : Fcn  Expr=cos(u)
  Gain : Gain  Gain=2/3  SaturateOnIntegerOverflow=on  OutDataTypeStr=Inherit: Same as input  ParamDataTypeStr=Inherit: Same as input
  Gain1 : Gain  Gain=2/3  SaturateOnIntegerOverflow=on  OutDataTypeStr=Inherit: Same as input  ParamDataTypeStr=Inherit: Same as input
  Mux : Mux  Inputs=[1 1 3]
  id : Fcn  Expr=u[1]*u[3]+(1.7320508*u[2]-u[1])*u[4]*0.5+(-u[1]-1.7320508*u[2])*u[5]*0.5
  iq : Fcn  Expr=-u[2]*u[3]+(u[2]+1.7320508*u[1])*u[4]*0.5+(u[2]-1.7320508*u[1])*u[5]*0.5
  Id : Outport  InitialOutput=0
  Iq : Outport  Port=2  InitialOutput=0
  wires:
  Fcn/1 -> Mux/2
  Fcn1/1 -> Mux/1
  Teta/1 -> Fcn1/1, Fcn/1
  Mux/1 -> iq/1, id/1
  Iabc/1 -> Mux/3
  iq/1 -> Gain1/1
  id/1 -> Gain/1
  Gain/1 -> Id/1
  Gain1/1 -> Iq/1

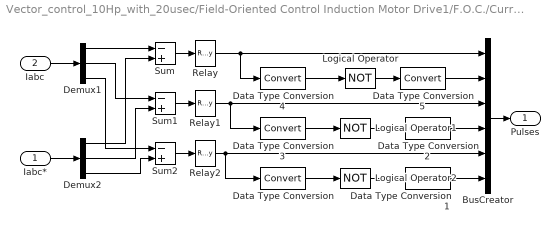
== system Vector_control_10Hp_with_20usec/Field-Oriented Control Induction Motor Drive1/F.O.C./Current Regulator ==
  Iabc* : Inport
  Iabc : Inport  Port=2
  BusCreator : BusCreator  Inputs=6
  Data Type Conversion{,1..5} (6 alike) : DataTypeConversion  SaturateOnIntegerOverflow=on  RndMeth=Zero
  Demux1 : Demux  Outputs=3
  Demux2 : Demux  Outputs=3
  Logical Operator : Logic  Operator=NOT
  Logical Operator1 : Logic  Operator=NOT
  Logical Operator2 : Logic  Operator=NOT
  Relay : Relay  OnSwitchValue=h/2  OffSwitchValue=-h/2
  Relay1 : Relay  OnSwitchValue=h/2  OffSwitchValue=-h/2
  Relay2 : Relay  OnSwitchValue=h/2  OffSwitchValue=-h/2
  Sum : Sum  Inputs=-+  SaturateOnIntegerOverflow=on  InputSameDT=on  OutDataTypeStr=Inherit: Same as first input
  Sum1 : Sum  Inputs=-+  SaturateOnIntegerOverflow=on  InputSameDT=on  OutDataTypeStr=Inherit: Same as first input
  Sum2 : Sum  Inputs=-+  SaturateOnIntegerOverflow=on  InputSameDT=on  OutDataTypeStr=Inherit: Same as first input
  Pulses : Outport  InitialOutput=0
  wires:
  Data Type Conversion5/1 -> BusCreator/2
  Data Type Conversion4/1 -> Logical Operator/1
  Data Type Conversion3/1 -> Logical Operator1/1
  Data Type Conversion2/1 -> BusCreator/4
  Data Type Conversion1/1 -> BusCreator/6
  Data Type Conversion/1 -> Logical Operator2/1
  Sum/1 -> Relay/1
  Sum1/1 -> Relay1/1
  Demux1/1 -> Sum/1
  Demux1/2 -> Sum1/1
  BusCreator/1 -> Pulses/1
  Iabc/1 -> Demux1/1
  Sum2/1 -> Relay2/1
  Demux1/3 -> Sum2/1
  Demux2/3 -> Sum2/2
  Demux2/2 -> Sum1/2
  Demux2/1 -> Sum/2
  Iabc*/1 -> Demux2/1
  Relay/1 -> Data Type Conversion4/1, BusCreator/1
  Relay1/1 -> Data Type Conversion3/1, BusCreator/3
  Relay2/1 -> Data Type Conversion/1, BusCreator/5
  Logical Operator/1 -> Data Type Conversion5/1
  Logical Operator1/1 -> Data Type Conversion2/1
  Logical Operator2/1 -> Data Type Conversion1/1

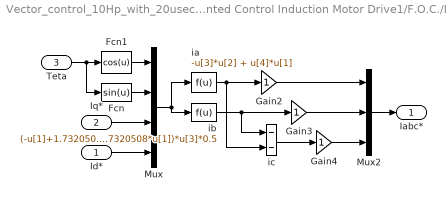
== system Vector_control_10Hp_with_20usec/Field-Oriented Control Induction Motor Drive1/F.O.C./DQ-ABC ==
  Id* : Inport
  Iq* : Inport  Port=2
  Teta : Inport  Port=3
  Fcn : Fcn  Expr=sin(u)
  Fcn1 : Fcn  Expr=cos(u)
  Gain2 : Gain  SaturateOnIntegerOverflow=on  OutDataTypeStr=Inherit: Same as input  ParamDataTypeStr=Inherit: Same as input
  Gain3 : Gain  SaturateOnIntegerOverflow=on  OutDataTypeStr=Inherit: Same as input  ParamDataTypeStr=Inherit: Same as input
  Gain4 : Gain  SaturateOnIntegerOverflow=on  OutDataTypeStr=Inherit: Same as input  ParamDataTypeStr=Inherit: Same as input
  Mux : Mux
  Mux2 : Mux  Inputs=3
  ia : Fcn  Expr=-u[3]*u[2] + u[4]*u[1]
  ib : Fcn  Expr=(-u[1]+1.7320508*u[2])*u[4]*0.5+(u[2]+1.7320508*u[1])*u[3]*0.5
  ic : Sum  Inputs=--  SaturateOnIntegerOverflow=on  InputSameDT=on  OutDataTypeStr=Inherit: Same as first input
  Iabc* : Outport  InitialOutput=0
  wires:
  Fcn/1 -> Mux/2
  Fcn1/1 -> Mux/1
  Mux2/1 -> Iabc*/1
  Mux/1 -> ib/1, ia/1
  Teta/1 -> Fcn1/1, Fcn/1
  Iq*/1 -> Mux/3
  Id*/1 -> Mux/4
  Gain3/1 -> Mux2/2
  ic/1 -> Gain4/1
  Gain4/1 -> Mux2/3
  Gain2/1 -> Mux2/1
  ia/1 -> Gain2/1, ic/2
  ib/1 -> Gain3/1, ic/1

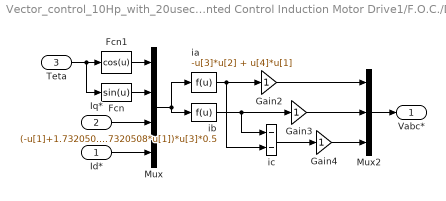
== system Vector_control_10Hp_with_20usec/Field-Oriented Control Induction Motor Drive1/F.O.C./DQ-ABC1 ==
  Id* : Inport
  Iq* : Inport  Port=2
  Teta : Inport  Port=3
  Fcn : Fcn  Expr=sin(u)
  Fcn1 : Fcn  Expr=cos(u)
  Gain2 : Gain  SaturateOnIntegerOverflow=on  OutDataTypeStr=Inherit: Same as input  ParamDataTypeStr=Inherit: Same as input
  Gain3 : Gain  SaturateOnIntegerOverflow=on  OutDataTypeStr=Inherit: Same as input  ParamDataTypeStr=Inherit: Same as input
  Gain4 : Gain  SaturateOnIntegerOverflow=on  OutDataTypeStr=Inherit: Same as input  ParamDataTypeStr=Inherit: Same as input
  Mux : Mux
  Mux2 : Mux  Inputs=3
  ia : Fcn  Expr=-u[3]*u[2] + u[4]*u[1]
  ib : Fcn  Expr=(-u[1]+1.7320508*u[2])*u[4]*0.5+(u[2]+1.7320508*u[1])*u[3]*0.5
  ic : Sum  Inputs=--  SaturateOnIntegerOverflow=on  InputSameDT=on  OutDataTypeStr=Inherit: Same as first input
  Vabc* : Outport  InitialOutput=0
  wires:
  ib/1 -> ic/1, Gain3/1
  ia/1 -> ic/2, Gain2/1
  Gain2/1 -> Mux2/1
  Gain4/1 -> Mux2/3
  ic/1 -> Gain4/1
  Gain3/1 -> Mux2/2
  Id*/1 -> Mux/4
  Iq*/1 -> Mux/3
  Teta/1 -> Fcn/1, Fcn1/1
  Mux/1 -> ia/1, ib/1
  Mux2/1 -> Vabc*/1
  Fcn1/1 -> Mux/1
  Fcn/1 -> Mux/2

== system Vector_control_10Hp_with_20usec/Field-Oriented Control Induction Motor Drive1/F.O.C./Flux Calculation ==
  note: Phir = Lm *Id / (1 +Tr .s)
  Id : Inport
  Discrete Transfer Fcn1 : DiscreteTransferFcn  Numerator=[1-exp(-(Rr/(Lr))*Tvect)]  Denominator=[1 -exp(-(Rr/(Lr))*Tvect)]  SampleTime=Tvect
  Lm : Gain  Gain=Lm  SaturateOnIntegerOverflow=on  OutDataTypeStr=Inherit: Same as input  ParamDataTypeStr=Inherit: Same as input
  Phir : Outport
  wires:
  Discrete Transfer Fcn1/1 -> Phir/1
  Id/1 -> Lm/1
  Lm/1 -> Discrete Transfer Fcn1/1

== system Vector_control_10Hp_with_20usec/Field-Oriented Control Induction Motor Drive1/F.O.C./Flux_PI ==
  m_Flux : Inport
  Flux* : Inport  Port=2
  Discrete Transfer Fcn1 : DiscreteTransferFcn  Numerator=[1-exp(-(2*pi*20)*Tvect)]  Denominator=[1 -exp(-(2*pi*20)*Tvect)]  SampleTime=Tvect
  Discrete-Time Integrator : DiscreteIntegrator  IntegratorMethod=Integration: Trapezoidal  SampleTime=Tvect  LimitOutput=on  UpperSaturationLimit=csat(2)  LowerSaturationLimit=csat(1)  ICPrevOutput=DiscIntNeverNeededParam  ICPrevScaledInput=DiscIntNeverNeededParam
  Ki1 : Gain  Gain=ki  SaturateOnIntegerOverflow=on  OutDataTypeStr=Inherit: Same as input  ParamDataTypeStr=Inherit: Same as input
  Kp : Gain  Gain=kp  SaturateOnIntegerOverflow=on  OutDataTypeStr=Inherit: Same as input  ParamDataTypeStr=Inherit: Same as input
  Saturation : Saturate  UpperLimit=csat(2)  LowerLimit=csat(1)
  Sum : Sum  Inputs=|+-  SaturateOnIntegerOverflow=on
  Sum1 : Sum  Inputs=|++  SaturateOnIntegerOverflow=on
  Phir* : Outport
  wires:
  Sum/1 -> Kp/1, Ki1/1
  Discrete-Time Integrator/1 -> Sum1/1
  Kp/1 -> Sum1/2
  Sum1/1 -> Saturation/1
  Discrete Transfer Fcn1/1 -> Sum/2
  Flux*/1 -> Sum/1
  Saturation/1 -> Phir*/1
  m_Flux/1 -> Discrete Transfer Fcn1/1
  Ki1/1 -> Discrete-Time Integrator/1

== system Vector_control_10Hp_with_20usec/Field-Oriented Control Induction Motor Drive1/F.O.C./Flux_PI1 ==
  Id : Inport
  Id* : Inport  Port=2
  Discrete Transfer Fcn1 : DiscreteTransferFcn  Numerator=[1-exp(-(2*pi*200)*Tvect)]  Denominator=[1 -exp(-(2*pi*200)*Tvect)]  SampleTime=Tvect
  Discrete-Time Integrator : DiscreteIntegrator  IntegratorMethod=Integration: Trapezoidal  SampleTime=Tvect  LimitOutput=on  UpperSaturationLimit=321  LowerSaturationLimit=-321  ICPrevOutput=DiscIntNeverNeededParam  ICPrevScaledInput=DiscIntNeverNeededParam
  Ki1 : Gain  Gain=50  SaturateOnIntegerOverflow=on  OutDataTypeStr=Inherit: Same as input  ParamDataTypeStr=Inherit: Same as input
  Kp : Gain  Gain=50  SaturateOnIntegerOverflow=on  OutDataTypeStr=Inherit: Same as input  ParamDataTypeStr=Inherit: Same as input
  Saturation : Saturate  UpperLimit=321  LowerLimit=-321
  Sum : Sum  Inputs=|+-  SaturateOnIntegerOverflow=on
  Sum1 : Sum  Inputs=|++  SaturateOnIntegerOverflow=on
  Vd : Outport
  wires:
  Ki1/1 -> Discrete-Time Integrator/1
  Id/1 -> Discrete Transfer Fcn1/1
  Saturation/1 -> Vd/1
  Id*/1 -> Sum/1
  Discrete Transfer Fcn1/1 -> Sum/2
  Sum1/1 -> Saturation/1
  Kp/1 -> Sum1/2
  Discrete-Time Integrator/1 -> Sum1/1
  Sum/1 -> Ki1/1, Kp/1

== system Vector_control_10Hp_with_20usec/Field-Oriented Control Induction Motor Drive1/F.O.C./Flux_PI2 ==
  Iq : Inport
  Iq* : Inport  Port=2
  Discrete Transfer Fcn1 : DiscreteTransferFcn  Numerator=[1-exp(-(2*pi*200)*Tvect)]  Denominator=[1 -exp(-(2*pi*200)*Tvect)]  SampleTime=Tvect
  Discrete-Time Integrator : DiscreteIntegrator  IntegratorMethod=Integration: Trapezoidal  SampleTime=Tvect  LimitOutput=on  UpperSaturationLimit=321  LowerSaturationLimit=-321  ICPrevOutput=DiscIntNeverNeededParam  ICPrevScaledInput=DiscIntNeverNeededParam
  Ki1 : Gain  Gain=50  SaturateOnIntegerOverflow=on  OutDataTypeStr=Inherit: Same as input  ParamDataTypeStr=Inherit: Same as input
  Kp : Gain  Gain=50  SaturateOnIntegerOverflow=on  OutDataTypeStr=Inherit: Same as input  ParamDataTypeStr=Inherit: Same as input
  Saturation : Saturate  UpperLimit=321  LowerLimit=-321
  Sum : Sum  Inputs=|+-  SaturateOnIntegerOverflow=on
  Sum1 : Sum  Inputs=|++  SaturateOnIntegerOverflow=on
  Vq : Outport
  wires:
  Sum/1 -> Kp/1, Ki1/1
  Discrete-Time Integrator/1 -> Sum1/1
  Kp/1 -> Sum1/2
  Sum1/1 -> Saturation/1
  Discrete Transfer Fcn1/1 -> Sum/2
  Iq*/1 -> Sum/1
  Saturation/1 -> Vq/1
  Iq/1 -> Discrete Transfer Fcn1/1
  Ki1/1 -> Discrete-Time Integrator/1

== system Vector_control_10Hp_with_20usec/Field-Oriented Control Induction Motor Drive1/F.O.C./M_vector ==
  Constant1 : Constant  Value=[1 0 1 0 1 0]
  Constant3 : Constant  Value=[1 0 0 1 1 0]
  Demux : Demux  Outputs=6
  Pulse Generator1 : DiscretePulseGenerator  Period=8  PulseWidth=2  SampleTime=Tvect
  Scope : Scope
      settings: SaveName=ScopeData6
  Scope1 : Scope  NumInputPorts=6
      settings: YMin=-5~-5~-5~-5~-5~-5  YMax=5~5~5~5~5~5  SaveName=ScopeData7
  Switch1 : Switch  Threshold=0.5  SaturateOnIntegerOverflow=on
  Zero-Order Hold8 : ZeroOrderHold  SampleTime=Tvect
  vector : Outport
  wires:
  Constant3/1 -> Switch1/1
  Constant1/1 -> Switch1/3
  Pulse Generator1/1 -> Scope/1, Zero-Order Hold8/1
  Zero-Order Hold8/1 -> Switch1/2
  Switch1/1 -> Demux/1, vector/1
  Demux/6 -> Scope1/6
  Demux/3 -> Scope1/3
  Demux/4 -> Scope1/4
  Demux/2 -> Scope1/2
  Demux/5 -> Scope1/5
  Demux/1 -> Scope1/1

== system Vector_control_10Hp_with_20usec/Field-Oriented Control Induction Motor Drive1/F.O.C./Magnetisation ==
  Est_Flux : Inport
  Constant : Constant  Value=in_flux
  Constant1 : Constant  Value=0
  Data Type Conversion5 : DataTypeConversion  SaturateOnIntegerOverflow=on  RndMeth=Zero
  Relational Operator : RelationalOperator
  S-R Flip-Flop : simulink_extras/Flip Flops/S-R Flip-Flop  initial_condition=0
  Terminator : Terminator
  Zero-Order Hold5 : ZeroOrderHold  SampleTime=Tvect
  Start : Outport
  wires:
  Data Type Conversion5/1 -> S-R Flip-Flop/2
  Est_Flux/1 -> Relational Operator/1
  Relational Operator/1 -> S-R Flip-Flop/1
  Constant/1 -> Zero-Order Hold5/1
  Constant1/1 -> Data Type Conversion5/1
  S-R Flip-Flop/1 -> Start/1
  S-R Flip-Flop/2 -> Terminator/1
  Zero-Order Hold5/1 -> Relational Operator/2

== system Vector_control_10Hp_with_20usec/Field-Oriented Control Induction Motor Drive1/F.O.C./Switching control ==
  Pulses : Inport
  Control 1-2 : Subsystem
  Control 3-4 : Subsystem
  Control 5-6 : Subsystem
  Demux : Demux  Outputs=6
  Mux : Mux  Inputs=6
  RF Pulses : Outport
  wires:
  Control 5-6/2(!S_Limited) -> Mux/6
  Control 5-6/1(S_Limited) -> Mux/5
  Control 3-4/2(!S_Limited) -> Mux/4
  Control 3-4/1(S_Limited) -> Mux/3
  Control 1-2/2(!S_Limited) -> Mux/2
  Control 1-2/1(S_Limited) -> Mux/1
  Demux/6 -> Control 5-6/2(!S)
  Demux/5 -> Control 5-6/1(S)
  Demux/4 -> Control 3-4/2(!S)
  Demux/3 -> Control 3-4/1(S)
  Demux/2 -> Control 1-2/2(!S)
  Demux/1 -> Control 1-2/1(S)
  Mux/1 -> RF Pulses/1
  Pulses/1 -> Demux/1

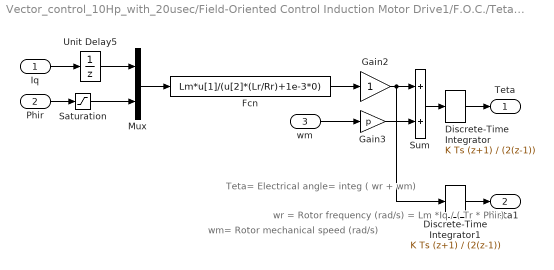
== system Vector_control_10Hp_with_20usec/Field-Oriented Control Induction Motor Drive1/F.O.C./Teta Calculation ==
  note: Teta= Electrical angle= integ ( wr + wm)
  note: wr = Rotor frequency (rad/s) = Lm *Iq / ( Tr * Phir)
  note: wm= Rotor mechanical speed (rad/s)
  Iq : Inport
  Phir : Inport  Port=2
  wm : Inport  Port=3
  Discrete-Time Integrator : DiscreteIntegrator  IntegratorMethod=Integration: Trapezoidal  SampleTime=Tvect  ICPrevOutput=DiscIntNeverNeededParam  ICPrevScaledInput=DiscIntNeverNeededParam
  Discrete-Time Integrator1 : DiscreteIntegrator  IntegratorMethod=Integration: Trapezoidal  SampleTime=Tvect  ICPrevOutput=DiscIntNeverNeededParam  ICPrevScaledInput=DiscIntNeverNeededParam
  Fcn : Fcn  Expr=Lm*u[1]/(u[2]*(Lr/Rr)+1e-3*0)
  Gain2 : Gain  SaturateOnIntegerOverflow=on  OutDataTypeStr=Inherit: Same as input  ParamDataTypeStr=Inherit: Same as input
  Gain3 : Gain  Gain=p  SaturateOnIntegerOverflow=on  OutDataTypeStr=Inherit: Same as input  ParamDataTypeStr=Inherit: Same as input
  Mux : Mux  Inputs=2
  Saturation : Saturate  UpperLimit=inf  LowerLimit=1e-3
  Sum : Sum  SaturateOnIntegerOverflow=on  InputSameDT=on  OutDataTypeStr=Inherit: Same as first input
  Unit Delay5 : UnitDelay  SampleTime=Tvect
  Teta : Outport  InitialOutput=0
  Teta1 : Outport  Port=2  InitialOutput=0
  wires:
  Discrete-Time Integrator/1 -> Teta/1
  Sum/1 -> Discrete-Time Integrator/1
  Gain3/1 -> Sum/2
  wm/1 -> Gain3/1
  Fcn/1 -> Gain2/1
  Phir/1 -> Saturation/1
  Iq/1 -> Unit Delay5/1
  Mux/1 -> Fcn/1
  Saturation/1 -> Mux/2
  Unit Delay5/1 -> Mux/1
  Discrete-Time Integrator1/1 -> Teta1/1
  Gain2/1 -> Discrete-Time Integrator1/1, Sum/1

== system Vector_control_10Hp_with_20usec/Field-Oriented Control Induction Motor Drive1/F.O.C./id* Calculation ==
  note: Id* = Phir*/ Lm
  note: Lm= 34.7 mH
  Phir* : Inport
  KF : Gain  Gain=1/Lm  SaturateOnIntegerOverflow=on  OutDataTypeStr=Inherit: Same as input  ParamDataTypeStr=Inherit: Same as input
  Id* : Outport
  wires:
  KF/1 -> Id*/1
  Phir*/1 -> KF/1

== system Vector_control_10Hp_with_20usec/Field-Oriented Control Induction Motor Drive1/F.O.C./iqs* Calculation ==
  Te* : Inport
  Phir : Inport  Port=2
  Fcn : Fcn  Expr=(2/3)*(1/p)*(Lr/Lm)*u[1]/(u[2]+1e-3*0)
  Mux1 : Mux  Inputs=2
  Saturation : Saturate  UpperLimit=inf  LowerLimit=1e-3
  Iq* : Outport  InitialOutput=0
  wires:
  Phir/1 -> Saturation/1
  Fcn/1 -> Iq*/1
  Te*/1 -> Mux1/1
  Mux1/1 -> Fcn/1
  Saturation/1 -> Mux1/2

== system Vector_control_10Hp_with_20usec/Field-Oriented Control Induction Motor Drive1/Speed Controller/Flux table ==
  |N| : Inport
  Abs1 : Abs  SaturateOnIntegerOverflow=on
  F : Fcn  Expr=bs*nf/u(1)
  Saturation : Saturate  UpperLimit=inf  LowerLimit=bs
  Flux : Outport
  wires:
  Abs1/1 -> Saturation/1
  F/1 -> Flux/1
  |N|/1 -> Abs1/1
  Saturation/1 -> F/1

== system Vector_control_10Hp_with_20usec/Field-Oriented Control Induction Motor Drive1/F.O.C./Switching control/Control 1-2 ==
  S : Inport
  !S : Inport  Port=2
  Data Type Conversion2 : DataTypeConversion  OutDataTypeStr=boolean
  Data Type Conversion8 : DataTypeConversion  OutDataTypeStr=boolean
  Product2 : Product  RndMeth=Zero
  Product3 : Product  RndMeth=Zero
  S-R Flip-Flop1 : simulink_extras/Flip Flops/S-R Flip-Flop  initial_condition=0
  Subsystem1 : Subsystem
  Subsystem3 : Subsystem
  S_Limited : Outport
  !S_Limited : Outport  Port=2
  wires:
  !S/1 -> Product3/1
  S/1 -> Product2/2
  Subsystem1/1(Trig) -> Product3/2
  S-R Flip-Flop1/2 -> Subsystem1/1(Sig), !S_Limited/1
  Product3/1 -> Data Type Conversion8/1
  Data Type Conversion8/1 -> S-R Flip-Flop1/2
  Data Type Conversion2/1 -> S-R Flip-Flop1/1
  Subsystem3/1(Trig) -> Product2/1
  Product2/1 -> Data Type Conversion2/1
  S-R Flip-Flop1/1 -> Subsystem3/1(Sig), S_Limited/1

== system Vector_control_10Hp_with_20usec/Field-Oriented Control Induction Motor Drive1/F.O.C./Switching control/Control 3-4 ==
  S : Inport
  !S : Inport  Port=2
  Data Type Conversion2 : DataTypeConversion  OutDataTypeStr=boolean
  Data Type Conversion8 : DataTypeConversion  OutDataTypeStr=boolean
  Product2 : Product  RndMeth=Zero
  Product3 : Product  RndMeth=Zero
  S-R Flip-Flop1 : simulink_extras/Flip Flops/S-R Flip-Flop  initial_condition=0
  Subsystem1 : Subsystem
  Subsystem3 : Subsystem
  S_Limited : Outport
  !S_Limited : Outport  Port=2
  wires:
  S-R Flip-Flop1/1 -> S_Limited/1, Subsystem3/1(Sig)
  Product2/1 -> Data Type Conversion2/1
  Subsystem3/1(Trig) -> Product2/1
  Data Type Conversion2/1 -> S-R Flip-Flop1/1
  Data Type Conversion8/1 -> S-R Flip-Flop1/2
  Product3/1 -> Data Type Conversion8/1
  S-R Flip-Flop1/2 -> !S_Limited/1, Subsystem1/1(Sig)
  Subsystem1/1(Trig) -> Product3/2
  S/1 -> Product2/2
  !S/1 -> Product3/1

== system Vector_control_10Hp_with_20usec/Field-Oriented Control Induction Motor Drive1/F.O.C./Switching control/Control 5-6 ==
  S : Inport
  !S : Inport  Port=2
  Data Type Conversion2 : DataTypeConversion  OutDataTypeStr=boolean
  Data Type Conversion8 : DataTypeConversion  OutDataTypeStr=boolean
  Product2 : Product  RndMeth=Zero
  Product3 : Product  RndMeth=Zero
  S-R Flip-Flop1 : simulink_extras/Flip Flops/S-R Flip-Flop  initial_condition=0
  Subsystem1 : Subsystem
  Subsystem3 : Subsystem
  S_Limited : Outport
  !S_Limited : Outport  Port=2
  wires:
  !S/1 -> Product3/1
  S/1 -> Product2/2
  Subsystem1/1(Trig) -> Product3/2
  S-R Flip-Flop1/2 -> Subsystem1/1(Sig), !S_Limited/1
  Product3/1 -> Data Type Conversion8/1
  Data Type Conversion8/1 -> S-R Flip-Flop1/2
  Data Type Conversion2/1 -> S-R Flip-Flop1/1
  Subsystem3/1(Trig) -> Product2/1
  Product2/1 -> Data Type Conversion2/1
  S-R Flip-Flop1/1 -> Subsystem3/1(Sig), S_Limited/1

== system Vector_control_10Hp_with_20usec/Field-Oriented Control Induction Motor Drive1/F.O.C./Switching control/Control 1-2/Subsystem1 ==
  Sig : Inport
  Constant : Constant
  Constant1 : Constant  Value=freq_max
  Discrete-Time Integrator : DiscreteIntegrator  IntegratorMethod=Integration: Trapezoidal  ExternalReset=rising  SampleTime=Tvect  ICPrevOutput=DiscIntNeverNeededParam  ICPrevScaledInput=DiscIntNeverNeededParam
  Relational Operator : RelationalOperator  ZeroCross=off
  Unit Delay : UnitDelay  SampleTime=Tvect
  Trig : Outport
  wires:
  Unit Delay/1 -> Trig/1
  Sig/1 -> Discrete-Time Integrator/2
  Relational Operator/1 -> Unit Delay/1
  Discrete-Time Integrator/1 -> Relational Operator/1
  Constant/1 -> Relational Operator/2
  Constant1/1 -> Discrete-Time Integrator/1

== system Vector_control_10Hp_with_20usec/Field-Oriented Control Induction Motor Drive1/F.O.C./Switching control/Control 1-2/Subsystem3 ==
  Sig : Inport
  Constant : Constant
  Constant1 : Constant  Value=freq_max
  Discrete-Time Integrator : DiscreteIntegrator  IntegratorMethod=Integration: Trapezoidal  ExternalReset=rising  SampleTime=Tvect  ICPrevOutput=DiscIntNeverNeededParam  ICPrevScaledInput=DiscIntNeverNeededParam
  Relational Operator : RelationalOperator  ZeroCross=off
  Unit Delay : UnitDelay  SampleTime=Tvect
  Trig : Outport
  wires:
  Constant1/1 -> Discrete-Time Integrator/1
  Constant/1 -> Relational Operator/2
  Discrete-Time Integrator/1 -> Relational Operator/1
  Relational Operator/1 -> Unit Delay/1
  Sig/1 -> Discrete-Time Integrator/2
  Unit Delay/1 -> Trig/1

== system Vector_control_10Hp_with_20usec/Field-Oriented Control Induction Motor Drive1/F.O.C./Switching control/Control 3-4/Subsystem1 ==
  Sig : Inport
  Constant : Constant
  Constant1 : Constant  Value=freq_max
  Discrete-Time Integrator : DiscreteIntegrator  IntegratorMethod=Integration: Trapezoidal  ExternalReset=rising  SampleTime=Tvect  ICPrevOutput=DiscIntNeverNeededParam  ICPrevScaledInput=DiscIntNeverNeededParam
  Relational Operator : RelationalOperator  ZeroCross=off
  Unit Delay : UnitDelay  SampleTime=Tvect
  Trig : Outport
  wires:
  Constant1/1 -> Discrete-Time Integrator/1
  Constant/1 -> Relational Operator/2
  Discrete-Time Integrator/1 -> Relational Operator/1
  Relational Operator/1 -> Unit Delay/1
  Sig/1 -> Discrete-Time Integrator/2
  Unit Delay/1 -> Trig/1

== system Vector_control_10Hp_with_20usec/Field-Oriented Control Induction Motor Drive1/F.O.C./Switching control/Control 3-4/Subsystem3 ==
  Sig : Inport
  Constant : Constant
  Constant1 : Constant  Value=freq_max
  Discrete-Time Integrator : DiscreteIntegrator  IntegratorMethod=Integration: Trapezoidal  ExternalReset=rising  SampleTime=Tvect  ICPrevOutput=DiscIntNeverNeededParam  ICPrevScaledInput=DiscIntNeverNeededParam
  Relational Operator : RelationalOperator  ZeroCross=off
  Unit Delay : UnitDelay  SampleTime=Tvect
  Trig : Outport
  wires:
  Unit Delay/1 -> Trig/1
  Sig/1 -> Discrete-Time Integrator/2
  Relational Operator/1 -> Unit Delay/1
  Discrete-Time Integrator/1 -> Relational Operator/1
  Constant/1 -> Relational Operator/2
  Constant1/1 -> Discrete-Time Integrator/1

== system Vector_control_10Hp_with_20usec/Field-Oriented Control Induction Motor Drive1/F.O.C./Switching control/Control 5-6/Subsystem1 ==
  Sig : Inport
  Constant : Constant
  Constant1 : Constant  Value=freq_max
  Discrete-Time Integrator : DiscreteIntegrator  IntegratorMethod=Integration: Trapezoidal  ExternalReset=rising  SampleTime=Tvect  ICPrevOutput=DiscIntNeverNeededParam  ICPrevScaledInput=DiscIntNeverNeededParam
  Relational Operator : RelationalOperator  ZeroCross=off
  Unit Delay : UnitDelay  SampleTime=Tvect
  Trig : Outport
  wires:
  Unit Delay/1 -> Trig/1
  Sig/1 -> Discrete-Time Integrator/2
  Relational Operator/1 -> Unit Delay/1
  Discrete-Time Integrator/1 -> Relational Operator/1
  Constant/1 -> Relational Operator/2
  Constant1/1 -> Discrete-Time Integrator/1

== system Vector_control_10Hp_with_20usec/Field-Oriented Control Induction Motor Drive1/F.O.C./Switching control/Control 5-6/Subsystem3 ==
  Sig : Inport
  Constant : Constant
  Constant1 : Constant  Value=freq_max
  Discrete-Time Integrator : DiscreteIntegrator  IntegratorMethod=Integration: Trapezoidal  ExternalReset=rising  SampleTime=Tvect  ICPrevOutput=DiscIntNeverNeededParam  ICPrevScaledInput=DiscIntNeverNeededParam
  Relational Operator : RelationalOperator  ZeroCross=off
  Unit Delay : UnitDelay  SampleTime=Tvect
  Trig : Outport
  wires:
  Constant1/1 -> Discrete-Time Integrator/1
  Constant/1 -> Relational Operator/2
  Discrete-Time Integrator/1 -> Relational Operator/1
  Relational Operator/1 -> Unit Delay/1
  Sig/1 -> Discrete-Time Integrator/2
  Unit Delay/1 -> Trig/1
